simulink model "ilc_ramp"  (R2024a)
settings: Solver=ode45  StartTime=0.0  StopTime=2000  RelTol=1e-3  EnableMultiTasking=on
libraries: simulink_need_slupdate x1
settings Model: Creator=aeagr  LastModifiedBy=crcrisoft
settings SolverCC: AlgebraicLoopSolver=TrustRegion
settings DataIOCC: LimitDataPoints=on  SaveFormat=Array  SignalLoggingSaveFormat=ModelDataLogs  ReturnWorkspaceOutputs=off
settings OptimizationCC: ExpressionDepthLimit=2147483647  LifeSpan=inf
settings DebuggingCC: UnderspecifiedInitializationDetection=Classic  MergeDetectMultiDrivingBlocksExec=none  SolverPrmCheckMsg=warning  FcnCallInpInsideContextMsg=warning  UnconnectedInputMsg=warning  UnconnectedOutputMsg=warning  UnconnectedLineMsg=warning  StateNameClashWarn=warning  SFUnexpectedBacktrackingDiag=warning  SFNoUnconditionalDefaultTransitionDiag=warning  ArithmeticOperatorsInVariantConditions=warning
settings HardwareCC: ProdBitPerPointer=32  ProdBitPerSizeT=32  ProdBitPerPtrDiffT=32  ProdLargestAtomicFloat=None  ProdIntDivRoundTo=Undefined  ProdEndianess=Unspecified  ProdWordSize=32  ProdHWDeviceType=32-bit Generic
settings ModelReferenceCC: EnableRefExpFcnMdlSchedulingChecks=on  PropagateSignalLabelsOutOfModel=off
settings SFSimCC: SimUseLocalCustomCode=off  CustomCodeUndefinedFunction=UseInterfaceOnly
settings RTWCC: RTWUseLocalCustomCode=off  GPUComputeCapability=3.5
settings CodeAppCC: StateflowObjectComments=on
settings GRTTargetCC: TargetLangStandard=C89/C90 (ANSI)
settings ConfigComp: CovMetricSettings=dw  CovSaveCumulativeToWorkspaceVar=on  CovSaveSingleToWorkspaceVar=on  CovExternalEMLEnable=off

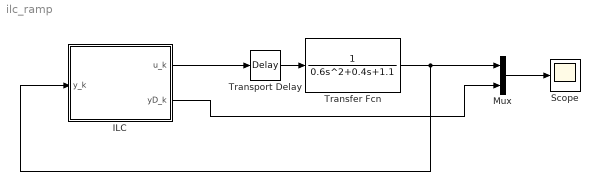
== system ilc_ramp ==
  ILC : Subsystem  Description=Iterative Learning Control  TreatAsAtomicUnit=on  SystemSampleTime=dt  mask{Yseq=[zeros(1,30) 1:30 30*ones(1,30) 29:-1:0]/30, dt=1, gamma=0.2}
      mask prompts: Yseq "Target output sequence"; dt "Time step"; gamma "Learning rate"
  Mux : Mux  Inputs=2
  Scope : Scope
  Transfer Fcn : TransferFcn  Denominator=[0.6 0.4 1.1]
  Transport Delay : TransportDelay  DelayTime=0.3
  wires:
  Transfer Fcn/1 -> ILC/1(y_k), Mux/1
  Mux/1 -> Scope/1
  ILC/2(yD_k) -> Mux/2
  ILC/1(u_k) -> Transport Delay/1
  Transport Delay/1 -> Transfer Fcn/1

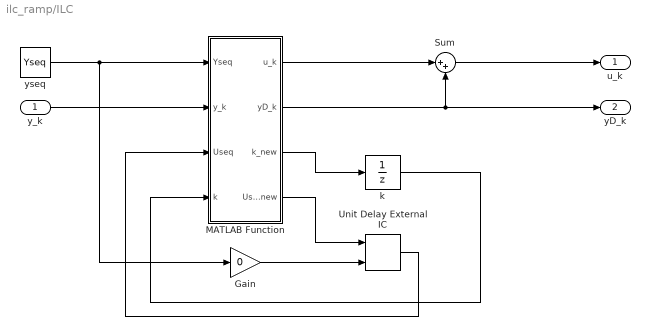
== system ilc_ramp/ILC ==
  y_k : Inport
  Gain : Gain  Gain=0
  MATLAB Function : MATLAB Function  TreatAsAtomicUnit=on
  Sum : Sum  Inputs=|++
  Unit Delay External IC : simulink_need_slupdate/Unit Delay External IC  tsamp=-1
  k : UnitDelay  InitialCondition=1  SampleTime=-1  HasFrameUpgradeWarning=on
  yseq : Constant  Value=Yseq
  u_k : Outport
  yD_k : Outport  Port=2
  wires:
  MATLAB Function/3(k_new) -> k/1
  MATLAB Function/4(Useq_new) -> Unit Delay External IC/1
  Unit Delay External IC/1 -> MATLAB Function/3(Useq)
  y_k/1 -> MATLAB Function/2(y_k)
  yseq/1 -> MATLAB Function/1(Yseq), Gain/1
  k/1 -> MATLAB Function/4(k)
  MATLAB Function/2(yD_k) -> Sum/2, yD_k/1
  Sum/1 -> u_k/1
  MATLAB Function/1(u_k) -> Sum/1
  Gain/1 -> Unit Delay External IC/2

== matlab function ilc_ramp/ILC/MATLAB Function ==
  data: u_k output; Yseq input; yD_k output; y_k input; Useq input; k input; k_new output; Useq_new output; gamma parameter
function [u_k,yD_k,k_new,Useq_new] = fcn(Yseq,y_k,Useq,k,gamma)
%#codegen

% number of elements in sequence

Nseq = numel(Yseq);

% counter
k_new = k+1;
% reset if we've been round the sequence
if k_new>Nseq,
    k_new=1;
end

% extract current demand signal
yD_k = Yseq(k);

% and the current control
u_k = Useq(k);

% form the error
e_k = yD_k - y_k;

% copy the control sequence over
Useq_new = Useq;

% which entry to update
k_learn = k-1;
if k_learn<1,
    k_learn=Nseq;
end

% do the learning update
Useq_new(k_learn) = Useq_new(k_learn) + gamma*e_k;
